simulink model "Plant"  (R2020b)
settings: Solver=VariableStepAuto  StartTime=0.0  StopTime=10.0  RelTol=1e-3
model workspace (MAT data in the model file):
  MActual = Simulink.Parameter
  MActual.Value = 0
  MActual.DataType = 'auto'
  MActual.Dimensions = [1 1]
  q0 = Simulink.Parameter
  q0.Value = [0; 0; 0]
  q0.DataType = 'auto'
  q0.Dimensions = [3 1]
  qdot0 = Simulink.Parameter
  qdot0.Value = [0; 0; 0]
  qdot0.DataType = 'auto'
  qdot0.Dimensions = [3 1]
libraries: RRProbotLibrary x4
settings Model: ParameterArgumentNames=MActual,q0,qdot0  OrderedModelArguments=off  Creator=alons  LastModifiedBy=alons

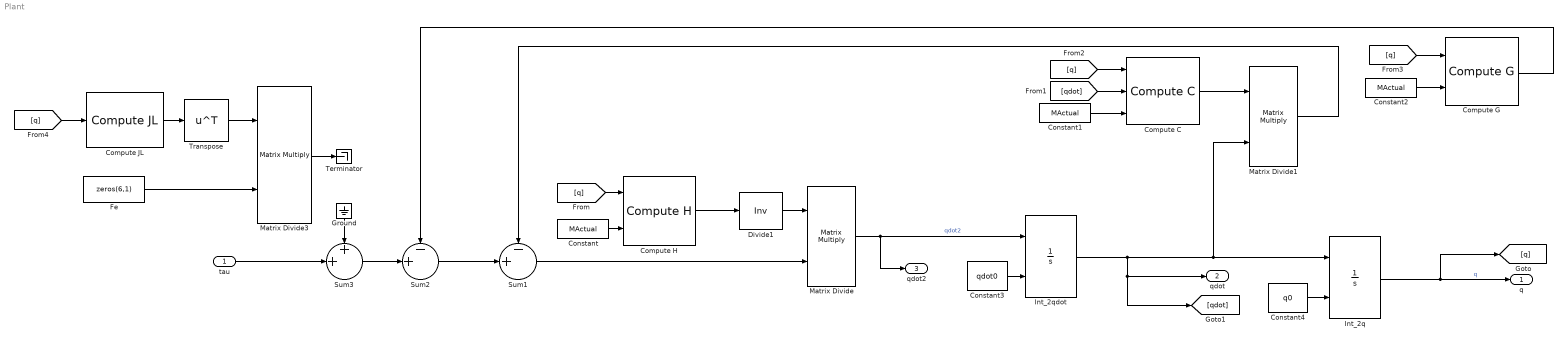
== system Plant ==
  tau : Inport  PortDimensions=3
  Compute C : RRProbotLibrary/Compute C  SystemSampleTime=-1  VariantActivationTime=update diagram  Latency=0  AutoFrameSizeCalculation=off
  Compute G : RRProbotLibrary/Compute G  SystemSampleTime=-1  VariantActivationTime=update diagram  Latency=0  AutoFrameSizeCalculation=off
  Compute H : RRProbotLibrary/Compute H  SystemSampleTime=-1  VariantActivationTime=update diagram  Latency=0  AutoFrameSizeCalculation=off
  Compute JL : RRProbotLibrary/Compute JL  SystemSampleTime=-1  VariantActivationTime=update diagram  Latency=0  AutoFrameSizeCalculation=off
  Constant : Constant  Value=MActual
  Constant1 : Constant  Value=MActual
  Constant2 : Constant  Value=MActual
  Constant3 : Constant  Value=qdot0
  Constant4 : Constant  Value=q0
  Divide1 : Product  Inputs=/  Multiplication=Matrix(*)
  Fe : Constant  Value=zeros(6,1)
  Ground : Ground
  Int_2q : Integrator  InitialConditionSource=external  InitialCondition=[0,0,0]'
  Int_2qdot : Integrator  InitialConditionSource=external  InitialCondition=[0,0,0]'
  Matrix Divide : Product  Inputs=**  Multiplication=Matrix(*)
  Matrix Divide1 : Product  Inputs=**  Multiplication=Matrix(*)
  Matrix Divide3 : Product  Inputs=**  Multiplication=Matrix(*)
  Sum1 : Sum  Inputs=-+|
  Sum2 : Sum  Inputs=-+|
  Sum3 : Sum  Inputs=++|
  Terminator : Terminator
  Transpose : Math  Operator=transpose  SaturateOnIntegerOverflow=on
  q : Outport
  qdot : Outport  Port=2
  qdot2 : Outport  Port=3
  wires:
  Matrix Divide1/1 -> Sum1/1
  tau/1 -> Sum3/2
  [q] -> Compute G/1
  [q] -> Compute JL/1
  Sum3/1 -> Sum2/2
  Compute JL/1 -> Transpose/1
  Transpose/1 -> Matrix Divide3/1
  [q] -> Compute H/1
  Matrix Divide/1 -> qdot2/1, Int_2qdot/1  "qdot2"
  Sum2/1 -> Sum1/2
  Compute H/1 -> Divide1/1
  Constant1/1 -> Compute C/3
  Int_2qdot/1 -> qdot/1, [qdot], Matrix Divide1/2, Int_2q/1
  Fe/1 -> Matrix Divide3/2
  Divide1/1 -> Matrix Divide/1
  Compute G/1 -> Sum2/1
  Constant/1 -> Compute H/2
  Ground/1 -> Sum3/1
  Compute C/1 -> Matrix Divide1/1
  Constant2/1 -> Compute G/2
  Int_2q/1 -> [q], q/1  "q"
  [qdot] -> Compute C/2
  [q] -> Compute C/1
  Matrix Divide3/1 -> Terminator/1
  Sum1/1 -> Matrix Divide/2
  Constant3/1 -> Int_2qdot/2
  Constant4/1 -> Int_2q/2
